simulink model "BLDC_1"  (R2015a)
settings: Solver=ode3  StartTime=0.0  StopTime=1.0  FixedStep=0.0000001  MaxStep=0.00001  MinStep=0.000001  RelTol=1e-3
libraries: powerlib x11, simulink x2
settings Model: Creator=hp  LastModifiedBy=hp

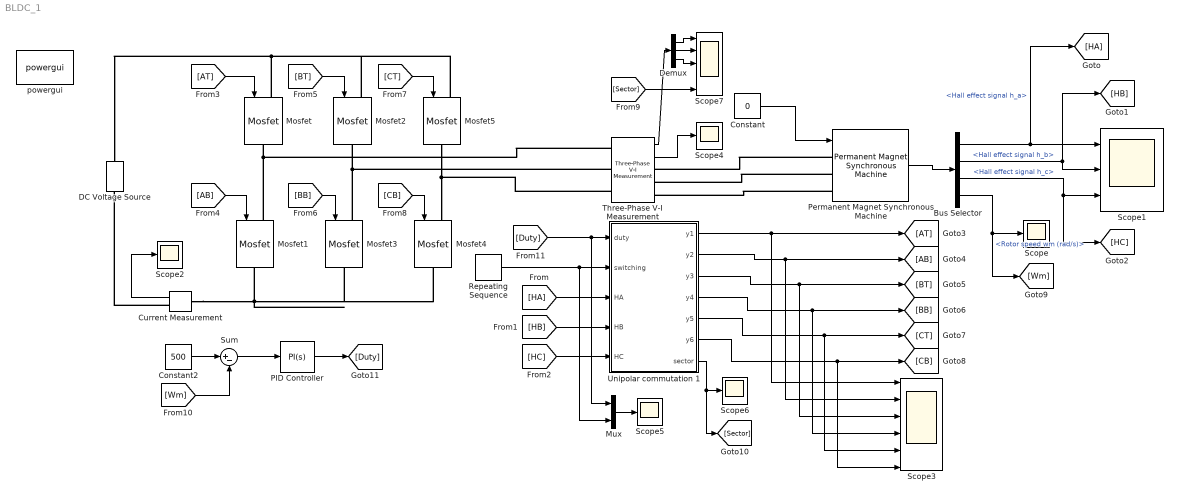
== system BLDC_1 ==
  Bus Selector : BusSelector  OutputSignals=Hall effect signal h_a,Hall effect signal h_b,Hall effect signal h_c,Rotor speed wm (rad/s)
  Constant : Constant  Value=0
  Constant2 : Constant  Value=500
  Current Measurement : powerlib/Measurements/Current Measurement  PhasorSimulation=off  OutputType=Complex  PSBequivalent=0
  DC Voltage Source : powerlib/Electrical Sources/DC Voltage Source  Amplitude=500  Measurements=None
  Demux : Demux  Outputs=3
  Mosfet{,1..5} (6 alike) : powerlib/Power Electronics/Mosfet  Ron=0.1  Lon=0  Rd=0.01  Vfd=0  IC=0  Rs=1e5  Cs=inf  Measurements=off
  Mux : Mux  Inputs=2
  PID Controller : simulink/Continuous/PID Controller  Controller=PI  TimeDomain=Continuous-time  SampleTime=-1  IntegratorMethod=Forward Euler  FilterMethod=Forward Euler  Form=Parallel  UseFilter=on  ControllerParametersSource=internal  P=0.01  I=0.1  D=0  N=100  InitialConditionSource=internal  InitialConditionForIntegrator=0  InitialConditionForFilter=0  ExternalReset=none  LimitOutput=off  UpperSaturationLimit=inf  LowerSaturationLimit=-inf  LinearizeAsGain=on  AntiWindupMode=none  Kb=1  TrackingMode=off  Kt=1  PParamMin=[]  PParamMax=[]  IParamMin=[]  IParamMax=[]  DParamMin=[]  DParamMax=[]  NParamMin=[]  NParamMax=[]  KbParamMin=[]  KbParamMax=[]  KtParamMin=[]  KtParamMax=[]  POutMin=[]  POutMax=[]  IOutMin=[]  IOutMax=[]  DOutMin=[]  DOutMax=[]  NOutMin=[]  NOutMax=[]  KbOutMin=[]  KbOutMax=[]  KtOutMin=[]  KtOutMax=[]  IntegratorOutMin=[]  IntegratorOutMax=[]  FilterOutMin=[]  FilterOutMax=[]  SumOutMin=[]  SumOutMax=[]  SumI1OutMin=[]  SumI1OutMax=[]  SumI2OutMin=[]  SumI2OutMax=[]  SumI3OutMin=[]  SumI3OutMax=[]  SumDOutMin=[]  SumDOutMax=[]  SaturationOutMin=[]  SaturationOutMax=[]  IntegratorContinuousStateAttributes=''  IntegratorStateMustResolveToSignalObject=off  IntegratorRTWStateStorageClass=Auto  FilterContinuousStateAttributes=''  FilterStateMustResolveToSignalObject=off  FilterRTWStateStorageClass=Auto  DifferentiatorICPrevScaledInput=0  DifferentiatorOutMin=[]  DifferentiatorOutMax=[]
  Permanent Magnet Synchronous Machine : powerlib/Machines/Permanent Magnet Synchronous Machine  NbPhases=3  FluxDistribution=Trapezoidal  RotorType=Round  MechanicalLoad=Torque Tm  PresetModel=No  ShowDetailedParameters=on  MeasurementBus=off  Resistance=0.0485  Inductance=8.5e-3  dqInductances=[8.5e-3,8.5e-3]  La=0.000395  MachineConstant=Flux linkage established by magnets (V.s)  Flux=0.1194  VoltageCst=100.0283  TorqueCst=0.9552  Flat=120  Mechanical=[0.0027 0.0004924 4 0]  PolePairs=4  InitialConditions=[0,0, 0,0]  InitialConditions5ph=[0 0 0 0 0 0]  TsPowergui=0  TsBlock=-1  RefAngle=Aligned with phase A axis (original Park)
  Repeating Sequence : simulink/Sources/Repeating Sequence  rep_seq_t=[0 1]/20000  rep_seq_y=[0 1]
  Scope{,2,4..6} (5 alike) : Scope
      Scope settings: YMin=-10  YMax=30
      Scope2 settings: YMin=0  YMax=7.5  SaveName=ScopeData2
      Scope4 settings: YMin=-100  YMax=100  SaveName=ScopeData4
      Scope5 settings: YMin=0  YMax=1  SaveName=ScopeData5
      Scope6 settings: YMin=3.8  YMax=4.2  SaveName=ScopeData6
  Scope1 : Scope  NumInputPorts=3
      settings: YMin=-2~-2~-2  YMax=2~2~2
  Scope3 : Scope  NumInputPorts=6
      settings: YMin=-1~0.95~-1~-1~0.95~-1  YMax=1~1.05~1~1~1.05~1  SaveName=ScopeData3
  Scope7 : Scope  NumInputPorts=5
      settings: YMin=-125~-125~-125~-1~3.8  YMax=125~125~125~1~4.2  SaveName=ScopeData7
  Sum : Sum  Inputs=|+-
  Three-Phase V-I Measurement : powerlib/Measurements/Three-Phase V-I Measurement  VoltageMeasurement=phase-to-phase  SetLabelV=off  LabelV=Vabc  Vpu=off  VpuLL=off  CurrentMeasurement=yes  SetLabelI=off  LabelI=Iabc  Ipu=off  Pbase=100e6  Vbase=500e3  OutputType=Complex  PhasorSimulation=off  PSBequivalent=0
  Unipolar commutation 1 : MATLAB Function  TreatAsAtomicUnit=on
  powergui : powerlib/powergui  Priority=1  SimulationMode=Continuous  SolverType=Tustin/Backward Euler (TBE)  SampleTime=1e-6  frequency=60  SPID=off  DisableSnubberDevices=off  DisableRonSwitches=off  DisableVfSwitches=off  SwTol=0  DisplayEquations=off  Interpol=off  methode=off  Ts=100  FunctionMessages=off  echomessages=off  HookPort=off  EnableUseOfTLC=off  x0status=blocks  frequencyindice=0  Pbase=100e6  ErrMax=1e-4  Iterations=50  UnitsV=kV  UnitsW=MW  buscounter=0  RestoreLinks=warning  ResistiveCurrentMeasurement=off  Frange=[0:2:500]  Ylog=off  Xlog=on  ShowGrid=off  save=off  variable=ZData  structure=0  ZoomFFT=off  StartTime=0.0  cycles=1  DisplayStyle=1  fundamental=60  FreqAxis=off  MaxFrequency=1000  frequencyindicesteady=1  RmsSteady=1  display=off
  wires:
  Constant/1 -> Permanent Magnet Synchronous Machine/1
  Permanent Magnet Synchronous Machine/1 -> Bus Selector/1
  Bus Selector/1 -> Scope1/1, [HA]  "<Hall effect signal h_a>"
  Bus Selector/2 -> Scope1/2, [HB]  "<Hall effect signal h_b>"
  Bus Selector/3 -> [HC], Scope1/3  "<Hall effect signal h_c>"
  [HA] -> Unipolar commutation 1/3(HA)
  [HB] -> Unipolar commutation 1/4(HB)
  [HC] -> Unipolar commutation 1/5(HC)
  Repeating Sequence/1 -> Unipolar commutation 1/2(switching), Mux/2
  Unipolar commutation 1/1(y1) -> Scope3/1, [AT]
  Unipolar commutation 1/2(y2) -> Scope3/2, [AB]
  Unipolar commutation 1/3(y3) -> Scope3/3, [BT]
  Unipolar commutation 1/4(y4) -> Scope3/4, [BB]
  Unipolar commutation 1/5(y5) -> Scope3/5, [CT]
  Unipolar commutation 1/6(y6) -> Scope3/6, [CB]
  [AT] -> Mosfet/1
  [AB] -> Mosfet1/1
  [BT] -> Mosfet2/1
  [BB] -> Mosfet3/1
  [CT] -> Mosfet5/1
  [CB] -> Mosfet4/1
  Bus Selector/4 -> [Wm], Scope/1  "<Rotor speed wm (rad/s)>"
  Current Measurement/1 -> Scope2/1
  Three-Phase V-I Measurement/2 -> Scope4/1
  Mux/1 -> Scope5/1
  Unipolar commutation 1/7(sector) -> [Sector], Scope6/1
  [Duty] -> Unipolar commutation 1/1(duty), Mux/1
  Three-Phase V-I Measurement/1 -> Demux/1
  [Sector] -> Scope7/5
  Demux/1 -> Scope7/1
  Demux/2 -> Scope7/2
  Demux/3 -> Scope7/3
  Constant2/1 -> Sum/1
  [Wm] -> Sum/2
  Sum/1 -> PID Controller/1
  PID Controller/1 -> [Duty]
  connections:
  Mosfet1/LConn1 -- Three-Phase V-I Measurement/LConn1 -- Mosfet/RConn1
  Mosfet4/RConn1 -- Mosfet3/RConn1 -- Current Measurement/LConn1 -- Mosfet1/RConn1
  Mosfet5/LConn1 -- Mosfet2/LConn1 -- DC Voltage Source/RConn1 -- Mosfet/LConn1
  Mosfet3/LConn1 -- Mosfet2/RConn1 -- Three-Phase V-I Measurement/LConn2
  Mosfet5/RConn1 -- Mosfet4/LConn1 -- Three-Phase V-I Measurement/LConn3
  Current Measurement/RConn1 -- DC Voltage Source/LConn1
  Permanent Magnet Synchronous Machine/LConn2 -- Three-Phase V-I Measurement/RConn2
  Permanent Magnet Synchronous Machine/LConn1 -- Three-Phase V-I Measurement/RConn1
  Permanent Magnet Synchronous Machine/LConn3 -- Three-Phase V-I Measurement/RConn3

== matlab function BLDC_1/Unipolar commutation 1 ==
  data: duty input; y1 output; switching input; HA input; HB input; HC input; y2 output; y3 output; y4 output; y5 output; y6 output; sector output
function [y1,y2,y3,y4,y5,y6,sector] = fcn(duty,switching, HA,HB,HC)
%#codegen
hall_state = (HA*4)+(HB*2)+(HC);
if hall_state==6                %sector 1
    if duty>switching           %V +ve W -ve
        y3 = 1;
        y1 = 0;
        y2 = 0;
        y4 = 0;
        y5 = 0;
    else
        y4 = 1;
        y1 = 0;
        y2 = 0;
        y3 = 0;
        y5 = 0;
    end
    y6 = 1;
    
elseif hall_state==2                %sector 2
    if duty>switching           %V +ve u -ve 
        y3 = 1;
        y1 = 0;
        y5 = 0;
        y6 = 0;
        y4 = 0;
    else
        y4 = 1;
        y1 = 0;
        y5 = 0;
        y6 = 0;
        y3 = 0;
    end
    y2 = 1;
elseif hall_state==3                %sector 3
    if duty>switching             %W +ve U -ve
        y5 = 1;
        y1 = 0;
        y3 = 0;
        y4 = 0;
        y6 = 0;
    else
        y6 = 1;
        y1 = 0;
        y3 = 0;
        y4 = 0;
        y5 = 0;
    end
    y2 = 1;
elseif hall_state==1                %sector 4
    if duty>switching           %W +ve V -ve
        y5 = 1;
        y1 = 0;
        y2 = 0;
        y3 = 0;
        y6 = 0;
    else
        y6 = 1;
        y1 = 0;
        y2 = 0;
        y3 = 0;
        y5 = 0;
    end
    y4 = 1;
elseif hall_state==5                %sector 5
    if duty>switching            %U +ve V -ve
        y1 = 1;
        y2 = 0;
        y3 = 0;
        y5 = 0;
        y6 = 0;
    else
        y2 = 1;
        y1 = 0;
        y3 = 0;
        y5 = 0;
        y6 = 0;
    end
    y4 = 1;
elseif hall_state==4                %sector 6
    if duty>switching             %U +ve W -ve
        y1 = 1;
        y2 = 0;
        y3 = 0;
        y4 = 0;
        y5 = 0;
    else
        y2 = 1;
        y1 = 0;
        y3 = 0;
        y4 = 0;
        y5 = 0;
    end
    y6 = 1;
else 
        y1 = 0;
        y2 = 0;
        y3 = 0;
        y4 = 0;
        y5 = 0;
        y6 = 0;
end    
sector = hall_state;
end
